simulink model "DC_motor_control"  (R2020b)
settings: Solver=VariableStepAuto  StartTime=0.0  StopTime=10.0  FixedStep=0.0000002  RelTol=1e-3
undefined symbols (not defined in the file or in its folder): b, j, k, Kd, Ki, Kp, L, r
settings Model: DataDictionary=DC_Motor_data.sldd  Creator=JAGRUTI SHINDE  LastModifiedBy=JAGRUTI SHINDE

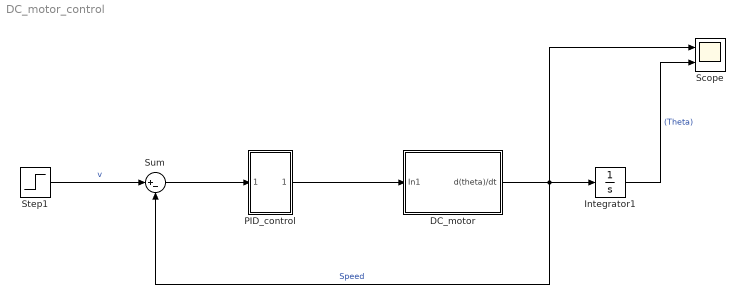
== system DC_motor_control ==
  DC_motor : Subsystem
  Integrator1 : Integrator
  PID_control : Subsystem
  Scope : Scope  NumInputPorts=2
  Step1 : Step  SampleTime=0
  Sum : Sum  Inputs=|+-
  wires:
  Step1/1 -> Sum/1  "v"
  DC_motor/1(d(theta)/dt) -> Scope/1, Integrator1/1, Sum/2  "Speed"
  Integrator1/1 -> Scope/2  "(Theta)"
  Sum/1 -> PID_control/1(In1)
  PID_control/1(Out1) -> DC_motor/1(In1)

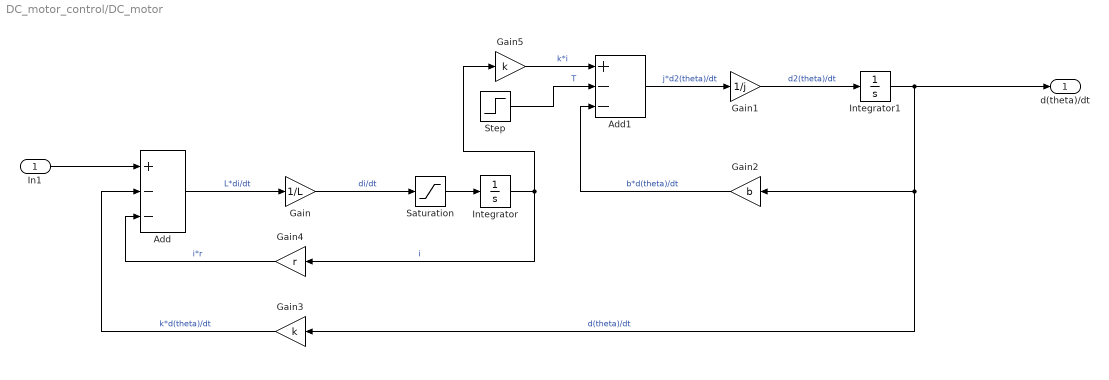
== system DC_motor_control/DC_motor ==
  In1 : Inport
  Add : Sum  Inputs=+--
  Add1 : Sum  Inputs=+--
  Gain : Gain  Gain=1/L
  Gain1 : Gain  Gain=1/j
  Gain2 : Gain  Gain=b
  Gain3 : Gain  Gain=k
  Gain4 : Gain  Gain=r
  Gain5 : Gain  Gain=k
  Integrator : Integrator
  Integrator1 : Integrator
  Saturation : Saturate
  Step : Step  After=-1  SampleTime=0
  d(theta)/dt : Outport
  wires:
  Integrator1/1 -> d(theta)/dt/1, Gain3/1, Gain2/1  "d(theta)/dt"
  Gain3/1 -> Add/2  "k*d(theta)/dt"
  Gain2/1 -> Add1/3  "b*d(theta)/dt"
  Step/1 -> Add1/2  "T"
  Gain1/1 -> Integrator1/1  "d2(theta)/dt"
  Gain4/1 -> Add/3  "i*r"
  Add/1 -> Gain/1  "L*di/dt"
  In1/1 -> Add/1
  Add1/1 -> Gain1/1  "j*d2(theta)/dt"
  Gain/1 -> Saturation/1  "di/dt"
  Gain5/1 -> Add1/1  "k*i"
  Integrator/1 -> Gain4/1, Gain5/1  "i"
  Saturation/1 -> Integrator/1

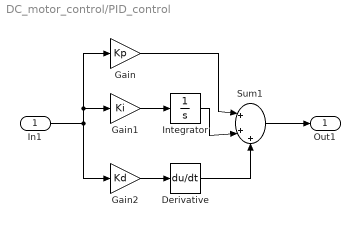
== system DC_motor_control/PID_control ==
  In1 : Inport
  Derivative : Derivative
  Gain : Gain  Gain=Kp
  Gain1 : Gain  Gain=Ki
  Gain2 : Gain  Gain=Kd
  Integrator : Integrator
  Sum1 : Sum  Inputs=|+++
  Out1 : Outport
  wires:
  Gain/1 -> Sum1/1
  In1/1 -> Gain1/1, Gain/1, Gain2/1
  Integrator/1 -> Sum1/2
  Derivative/1 -> Sum1/3
  Gain2/1 -> Derivative/1
  Sum1/1 -> Out1/1
  Gain1/1 -> Integrator/1
